simulink model "mpc_toolbox"  (R2020b)
settings: Solver=FixedStepAuto  StartTime=0.0  StopTime=0.1  FixedStep=0.001  RelTol=1e-3
InitFcn:
  | Lf = 0.6*10^-3;
  | Cf = 1338 * 10^-6;
  | Rf = 0.019;
  | RL = 2;
  | f_ac = 60;
  | f_sample = 20*10^3;
  | 
  | R_f = 19e-3;
  | L_f = 0.6e-3;
  | C_f = 1338e-6;
  | 
  | A = [0 1/C_f; -1/L_f -R_f/L_f];
  | B = [0 -1/C_f; 1/L_f 0];
  | C = [1 0; 1/RL 0];
  | D = zeros(2);
libraries: simulink x1, mpclib x1
settings Model: Creator=Kerim  LastModifiedBy=Kerim
settings SolverCC: ZeroCrossAlgorithm=Adaptive
settings DebuggingCC: IgnoredZcDiagnostic=none

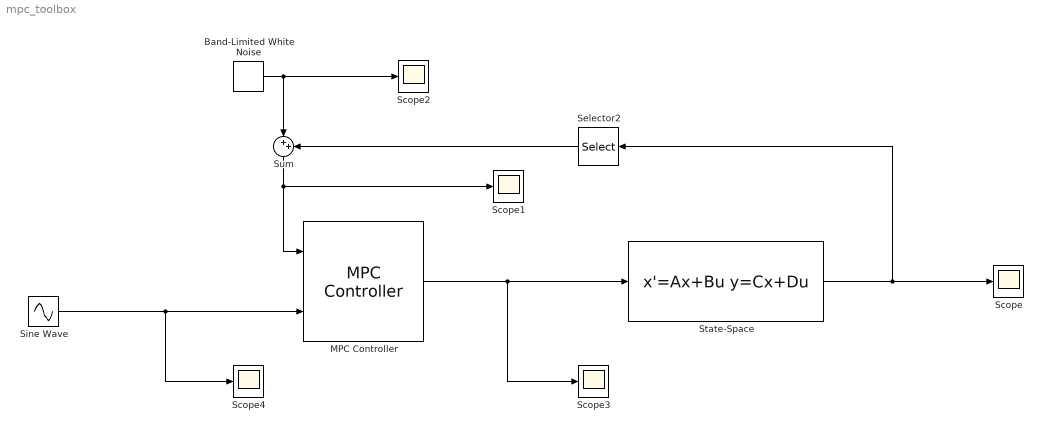
== system mpc_toolbox ==
  Band-Limited White Noise : simulink/Sources/Band-Limited White Noise  Cov=[0.5]  Ts=0.001  seed=[23341]
  MPC Controller : mpclib/MPC Controller  SCDEnableBlockLinearizationSpecification=on  mpcobj=mpc1  is_multiple=0  enable_value=0  return_u0=off  updateMPCinCallerWorkspace=on  md_inport=off  mv_inport=off  uref_inport=off  return_cost=off  return_mvseq=off  return_qpstatus=off  return_xseq=off  return_state=off  return_ovseq=off  state_inport=off  umin_inport=off  umax_inport=off  ymin_inport=off  ymax_inport=off  cc_inport=off  ywt_inport=off  uwt_inport=off  duwt_inport=off  rhoeps_inport=off  pm_inport=off  MaximumP=10  HorizonChoice=FixedHorizon  n_ts=0.001  n_p=1  n_mv=2  n_md=0  n_ud=0  n_mo=1  n_uo=0  BlockDataType=double  SampleTimeInherited=off  switch_inport=off
  Scope{,1..4} (5 alike) : Scope
  Selector2 : Selector  InputPortWidth=2  IndexOptions=Index vector (dialog)  Indices=[1]  OutputSizes=1
  Sine Wave : Sin  Amplitude=500  Frequency=f_ac * 2*pi  SampleTime=0
  State-Space : StateSpace  A=A  B=B  C=C  D=D  InitialCondition=0
  Sum : Sum  Inputs=|++
  wires:
  Sine Wave/1 -> MPC Controller/2, Scope4/1
  State-Space/1 -> Scope/1, Selector2/1
  Selector2/1 -> Sum/2
  Band-Limited White Noise/1 -> Scope2/1, Sum/1
  Sum/1 -> MPC Controller/1, Scope1/1
  MPC Controller/1 -> Scope3/1, State-Space/1
